simulink model "Hybrid_P2_Parallel"  (R2017b)
settings: Solver=FixedStepAuto  StartTime=0.0  StopTime=length(Speed)  FixedStep=0.01  MaxStep=0.01  RelTol=1e-3  EnableMultiTasking=on
PostLoadFcn:
  | , if any(exist('dsrtsu_mdlpostloadfcn', 'file') == [2, 3, 6]), try dsrtsu_mdlpostloadfcn('Execute', bdroot); catch fprintf('Error in PostLoadFcn (dsrtsu_mdlpostloadfcn) for model "%s":\n %s\n', bdroot, lasterr); end, end,
undefined symbols (not defined in the file): APP1_OOR, APP2_OOR, APP_Mismatch, Brk_Flt, cal, clt, Clutch, Clutch2, ClutchEngag, eng, Engine, EngOverTemp, ENGTRQ_MSMCH_Degraded_CP, ENGTRQ_MSMCH_ErrCritical_CP, ENGTRQ_MSMCH_LimpHome_CP, EngTrqMismatch, ess, ESSOverTemp, gb, KeyPos_Flt, LossCAN, MCUOverTemp, mot, MotDirMismatch, MotOverTemp, MotTrqMismatch, mph2kph, PRNDL_Flt, RegenFault, time, tloop
libraries: simulink x100, EC2_libraries x7, powerlib_meascontrol x2, lib_Actuators x1, CalculationGallon x1, lib_Chassis x1, autolibcoupling x1, autolibsharedcoupling x1, lib_DCDC x1, lib_Differential x1, lib_EMachine_2017a x1, lib_HVESS x1
(part 2 of 7)

== system Hybrid_P2_Parallel/Controller/HSC/Driver_Requests/APP_BPP to DrvIntndAxlTrq2 ==
  note: Note:Driver requested Axle Torque Calculation
  note: $Author: fy6949 $
      | $Rev: 577 $
      | $Date: 2017-1-19 08:53:15 -0500  $
  Sensors : Inport
  Diag : Inport  Port=2
  Controls : Inport  Port=3
  Bus Selector : BusSelector  OutputSignals=from_Analog.Driver_APP1,from_CAN.fromVEH_CAN.from_BCM.BrkPdlPos,from_CAN.fromEBCAN.from_ECM.VehSpdAvgDrvn,from_CAN.fromVEH_CAN.from_TCM.TrnGrRat,from_CAN.fromHV_CAN.from_MCU.INV_VCU_01.INV_Speed
  Bus Selector1 : BusSelector  OutputSignals=CompSig.RawSig.Driver_SigDiag.Drv_APP_Agree
  Bus Selector2 : BusSelector  OutputSignals=mode
  Post Driver Intnded Axle Torque : Subsystem
  Terminator : Terminator
  Terminator1 : Terminator
  IntndAxlTrq : Outport
  wires:
  Sensors/1 -> Bus Selector/1
  Controls/1 -> Bus Selector2/1
  Post Driver Intnded Axle Torque/1(IntndAxlTrq) -> IntndAxlTrq/1
  Bus Selector/2 -> Post Driver Intnded Axle Torque/2(BPP)  "<BrkPdlPos>"
  Bus Selector/3 -> Post Driver Intnded Axle Torque/3(VehicleSpeed)  "<VehSpdAvgDrvn>"
  Bus Selector/5 -> Post Driver Intnded Axle Torque/6(Motor_Speed)  "<INV_Speed>"
  Bus Selector/4 -> Post Driver Intnded Axle Torque/4(TransGearRatio)  "<TrnGrRat>"
  Bus Selector/1 -> Post Driver Intnded Axle Torque/1(APP)  "<Driver_APP1>"
  Post Driver Intnded Axle Torque/2(BrkIntndAxlTrq) -> Terminator/1
  Diag/1 -> Bus Selector1/1
  Bus Selector1/1 -> Terminator1/1  "<Drv_APP_Agree>"
  Bus Selector2/1 -> Post Driver Intnded Axle Torque/5(Mode)  "<mode>"

== system Hybrid_P2_Parallel/Controller/HSC/Powertrain Manager/Clutch Manager ==
  Sensors : Inport
  Control : Inport  Port=2
  Bus Creator : BusCreator  Inputs=2
  Bus Selector : BusSelector  OutputSignals=ClutchDisEngage
  Bus Selector1 : BusSelector  OutputSignals=from_CAN.fromEBCAN.from_CCU.CY01_posCurr,from_CAN.fromEBCAN.from_CCU.CY01_stMode,from_CAN.fromEBCAN.from_CCU.CY01_Counter,from_CAN.fromEBCAN.from_CCU.CY01_pCurr,from_CAN.fromHV_CAN.from_MCU.INV_VCU_01.INV_Speed,from_CAN.fromEBCAN.from_ECM.EngSpd,from_Analog.Driver_APP1,from_CAN.fromVEH_CAN.from_BCM.SysPwrMd,from_CAN.fromVEH_CAN.from_BCM.BrkPdlPos,from_CAN.fromVEH_CAN.from_TCM.TransEstGear
  Chart : Stateflow chart  Commented=on  TreatAsAtomicUnit=on
  Constant : Constant
  Constant1 : Constant  Value=2000
  Constant2 : Constant  Value=0
  Data Type Conversion : DataTypeConversion
  Switch : Switch  Criteria=u2 > Threshold
  Terminator{,1..9} (10 alike) : Terminator
  Out1 : Outport
  wires:
  Constant/1 -> Bus Creator/1  "MY15_CCU_stModeReq"
  Bus Creator/1 -> Out1/1
  Data Type Conversion/1 -> Bus Creator/2  "MY15_CCU_posDes"
  Control/1 -> Bus Selector/1
  Bus Selector/1 -> Switch/2  "<ClutchDisEngage>"
  Sensors/1 -> Bus Selector1/1
  Bus Selector1/1 -> Terminator/1  "<CY01_posCurr>"
  Bus Selector1/2 -> Terminator1/1  "<CY01_stMode>"
  Bus Selector1/3 -> Terminator2/1  "<CY01_Counter>"
  Bus Selector1/4 -> Terminator3/1  "<CY01_pCurr>"
  Bus Selector1/5 -> Terminator4/1  "<INV_Speed>"
  Bus Selector1/6 -> Terminator5/1  "<EngSpd>"
  Bus Selector1/7 -> Terminator6/1  "<Driver_APP1>"
  Bus Selector1/8 -> Terminator7/1  "<SysPwrMd>"
  Bus Selector1/9 -> Terminator8/1  "<BrkPdlPos>"
  Bus Selector1/10 -> Terminator9/1  "<TransEstGear>"
  Switch/1 -> Data Type Conversion/1
  Constant1/1 -> Switch/1
  Constant2/1 -> Switch/3

== system Hybrid_P2_Parallel/Controller/HSC/Powertrain Manager/HV Manager ==
  Sensors : Inport
  Controls : Inport  Port=2
  Axiomatic_Output_Manager : Subsystem
  BMS_Manager : Subsystem
  Bus Creator1 : BusCreator  Inputs=4
  DCDC Manager : Subsystem
  Invrter Manager : Subsystem
  OBC_Manager : Subsystem
  BMS_CAN : Outport
  HV_BUS_Status : Outport  Port=2
  OBC_CAN : Outport  Port=3
  OBC_Digital : Outport  Port=4
  BMS_Digital : Outport  Port=5
  Axiomatic_CAN : Outport  Port=6
  tag scope: MCU_CAN=global
  wires:
  Bus Creator1/1 -> [MCU_CAN]
  Invrter Manager/2(MCU_CAN) -> Bus Creator1/2  "MCU_CAN"
  Invrter Manager/1(MCU_Status) -> [MCU_Status], Bus Creator1/1  "MCU_Status"
  Sensors/1 -> BMS_Manager/1(Sensors), Invrter Manager/2(Sensors), DCDC Manager/1(BMSInput), Axiomatic_Output_Manager/1(Sensors), OBC_Manager/2(Sensors)
  [HV_BUS_Status] -> Invrter Manager/1(HV_Bus_Status)  "HV_BUS_Status"
  [HV_BUS_Status] -> Axiomatic_Output_Manager/2(HV_Bus_Status)
  BMS_Manager/2(HV_BUS_Status) -> [HV_BUS_Status], HV_BUS_Status/1  "HV_BUS_Status"
  [HV_BUS_Status] -> OBC_Manager/1(HV_Status)
  OBC_Manager/1(OBC CAN) -> OBC_CAN/1
  OBC_Manager/2(OBC_Digital) -> OBC_Digital/1
  Controls/1 -> BMS_Manager/2(Controls), Invrter Manager/3(Control), DCDC Manager/2(In1), DCDC Manager/3(In2)
  BMS_Manager/1(BMS CAN) -> BMS_CAN/1
  BMS_Manager/3(BMS Digital) -> BMS_Digital/1
  Axiomatic_Output_Manager/1(Axiomatic_CAN) -> Axiomatic_CAN/1
  Invrter Manager/3(MCU_Relay) -> Bus Creator1/3
  DCDC Manager/1(Out1) -> Bus Creator1/4
  [MCU_Status] -> BMS_Manager/3(In1)

== system Hybrid_P2_Parallel/Controller/HSC/Powertrain Manager/Output Conversion ==
  In1 : Inport
  In2 : Inport  Port=2
  In3 : Inport  Port=3
  In6 : Inport  Port=4
  In4 : Inport  Port=5
  In5 : Inport  Port=6
  In8 : Inport  Port=7
  In9 : Inport  Port=8
  In10 : Inport  Port=9
  In11 : Inport  Port=10
  Bus Creator : BusCreator  Inputs=14
  Bus Creator1 : BusCreator  Inputs=10
  Bus Selector2 : BusSelector  OutputSignals=powerMode,EnablePrplsn,ClutchDisEngage,EngAppReq,EngOnReq,MtrTrqCmd,EnableInverter,EngTrqCmd,HV_req,SysPwrMd_0_3,TransShftLvrPos,VehSpdAvgDrvn_kph,AccPos_Perc,SportsModeEnable
  Data Type Conversion{,2..3,5..13} (12 alike) : DataTypeConversion
  Memory : Memory
  Out1 : Outport
  wires:
  In10/1 -> Bus Creator1/9
  In9/1 -> Bus Creator1/8
  In8/1 -> Bus Creator1/7
  Memory/1 -> Data Type Conversion/1
  Data Type Conversion13/1 -> Bus Creator/13  "AccPos_Perc"
  Bus Selector2/13 -> Data Type Conversion13/1  "<AccPos_Perc>"
  Data Type Conversion12/1 -> Bus Creator/12  "VehSpdAvgDrvn_kph"
  Bus Selector2/12 -> Data Type Conversion12/1  "<VehSpdAvgDrvn_kph>"
  Data Type Conversion11/1 -> Bus Creator/11  "ShftLvrPos"
  Bus Selector2/11 -> Data Type Conversion11/1  "<TransShftLvrPos>"
  In5/1 -> Bus Creator1/6
  Bus Creator/1 -> Bus Creator1/5  "Controls"
  In3/1 -> Bus Creator1/3
  In2/1 -> Bus Creator1/2
  In1/1 -> Bus Creator1/1
  Bus Creator1/1 -> Out1/1
  Data Type Conversion5/1 -> Bus Creator/5  "EngOnReq"
  Data Type Conversion/1 -> Bus Creator/1  "powerMode"
  Data Type Conversion10/1 -> Bus Creator/10  "SysPwrMd"
  Data Type Conversion9/1 -> Bus Creator/9  "HV_req"
  Data Type Conversion8/1 -> Bus Creator/8  "EngTrqCmd"
  Data Type Conversion7/1 -> Bus Creator/7  "Inverter_Enable"
  Data Type Conversion6/1 -> Bus Creator/6  "Torque_Command"
  Bus Selector2/4 -> Bus Creator/4  "<EngAppReq>"
  Data Type Conversion3/1 -> Bus Creator/3  "ClutchDisEngage"
  Data Type Conversion2/1 -> Bus Creator/2  "EnablePrplsn"
  Bus Selector2/10 -> Data Type Conversion10/1  "<SysPwrMd_0_3>"
  Bus Selector2/9 -> Data Type Conversion9/1  "<HV_req>"
  Bus Selector2/8 -> Data Type Conversion8/1  "<EngTrqCmd>"
  Bus Selector2/7 -> Data Type Conversion7/1  "<EnableInverter>"
  Bus Selector2/6 -> Data Type Conversion6/1  "<MtrTrqCmd>"
  Bus Selector2/5 -> Data Type Conversion5/1  "<EngOnReq>"
  Bus Selector2/3 -> Data Type Conversion3/1  "<ClutchDisEngage>"
  Bus Selector2/2 -> Data Type Conversion2/1  "<EnablePrplsn>"
  Bus Selector2/1 -> Memory/1  "<powerMode>"
  In4/1 -> Bus Selector2/1
  In11/1 -> Bus Creator1/10
  Bus Selector2/14 -> Bus Creator/14  "<SportsModeEnable>"
  In6/1 -> Bus Creator1/4

== system Hybrid_P2_Parallel/Controller/HSC/Powertrain Manager/Thermal Manager ==
  In2 : Inport
  Bus Creator : BusCreator  Inputs=3
  Bus Creator1 : BusCreator  Inputs=4
  Bus Creator2 : BusCreator  Inputs=4
  Bus Creator3 : BusCreator  Inputs=3
  Bus Creator4 : BusCreator  Inputs=1
  Bus Selector : BusSelector  OutputSignals=from_CAN.fromEBCAN.from_ECM.EngCltTmp,from_CAN.fromHV_CAN.from_BMSHybrid.BMS_Temperatur,from_CAN.fromHV_CAN.from_MCU.INV_VCU_04.INV_InverterTemperature,from_CAN.fromHV_CAN.from_MCU.INV_VCU_04.INV_ElectricMachineTemperature,from_CAN.fromEBCAN.from_ECM.EngRunAtv,from_CAN.fromHV_CAN.from_BMSHybrid.BMS_HYB_02.BMS_IstModus,from_CAN.fromVEH_CAN.from_BCM.SysPwrMd,from_CAN.fromEBCAN.from_ECM.VehSpdAvgDrvn
  Bus Selector3 : BusSelector  OutputSignals=from_CAN.fromHV_CAN.from_BMSHybrid.BMS_HYB_02.BMS_Fehler_Pilot
  Compare To Constant1 : simulink/Logic and Bit Operations/Compare To Constant  relop=>  const=0  OutDataTypeStr=boolean
  Cooling Fan Manger : Subsystem
  Data Type Conversion : DataTypeConversion  OutDataTypeStr=double
  ESS Pump Manger : Subsystem
  MotInv Pump Manger : Subsystem
  Out1 : Outport
  wires:
  Bus Selector/8 -> Bus Creator/3  "<VehSpdAvgDrvn>"
  Bus Selector/7 -> Bus Creator3/3  "<SysPwrMd>"
  Bus Selector/6 -> Bus Creator3/2  "<BMS_IstModus>"
  Bus Selector/5 -> Bus Creator3/1  "<EngRunAtv>"
  Bus Selector/4 -> Bus Creator2/4  "<INV_ElectricMachineTemperature>"
  Bus Selector/3 -> Bus Creator2/3  "<INV_InverterTemperature>"
  Bus Selector/2 -> Bus Creator2/2  "<BMS_Temperatur>"
  Bus Selector/1 -> Bus Creator2/1  "<EngCltTmp>"
  Bus Creator1/1 -> Out1/1  "Thermal_Control"
  Cooling Fan Manger/1(Fan_control) -> Bus Creator1/1  "Fan_Control"
  Bus Creator/1 -> Cooling Fan Manger/1(Temp), ESS Pump Manger/1(ESS_temp), MotInv Pump Manger/1(MotInv_temp)
  ESS Pump Manger/1(ESS_Thermal_Control) -> Bus Creator1/2  "ESS_Pump_Control"
  MotInv Pump Manger/1(MotInvpump_control) -> Bus Creator1/3  "MotMCU_Pump_Control"
  Bus Creator2/1 -> Bus Creator/1  "Temp_Signals"
  Bus Creator3/1 -> Bus Creator/2  "Component_State"
  In2/1 -> Bus Selector3/1, Bus Selector/1
  Bus Selector3/1 -> Compare To Constant1/1  "<BMS_Fehler_Pilot>"
  Bus Creator4/1 -> Bus Creator1/4  "Pump_Commands"
  Data Type Conversion/1 -> Bus Creator4/1  "FuelPump_Disable"
  Compare To Constant1/1 -> Data Type Conversion/1

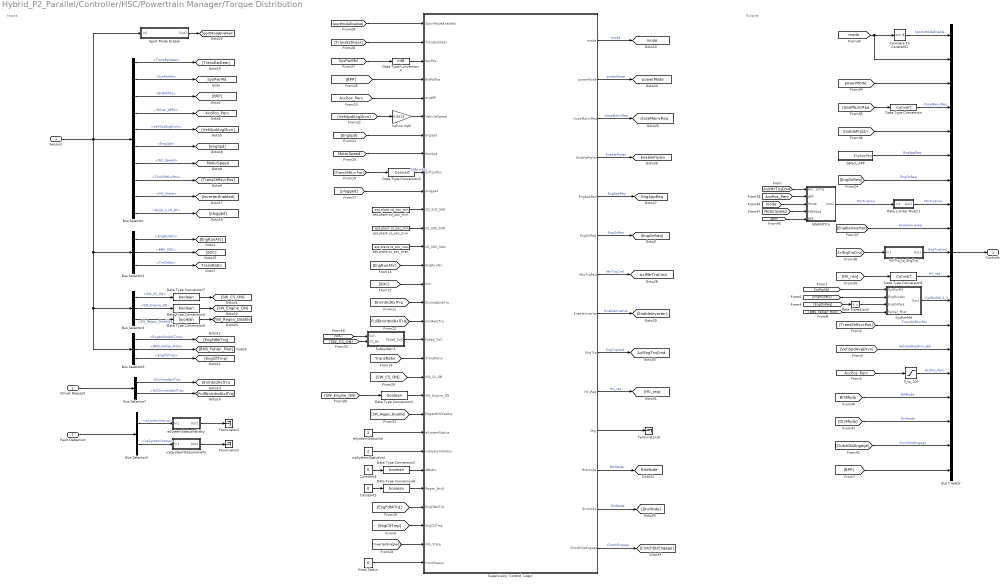
== system Hybrid_P2_Parallel/Controller/HSC/Powertrain Manager/Torque Distribution ==
  note: Inputs
  note: Outputs
  Sensors : Inport
  Driver Request : Inport  Port=2
  Fault Detection : Inport  Port=3
  0_to_100 : Saturate  UpperLimit=100  LowerLimit=0
  AxlTrq_to_EngTrq : Subsystem
  Bus Creator : BusCreator  Inputs=19
  Bus Selector : BusSelector  OutputSignals=from_CAN.fromVEH_CAN.from_TCM.TransEstGear,from_CAN.fromVEH_CAN.from_BCM.SysPwrMd,from_CAN.fromVEH_CAN.from_BCM.BrkPdlPos,from_Analog.Driver_APP1,from_CAN.fromEBCAN.from_ECM.VehSpdAvgDrvn,from_CAN.fromEBCAN.from_ECM.EngSpd,from_CAN.fromHV_CAN.from_MCU.INV_VCU_01.INV_Speed,from_CAN.fromVEH_CAN.from_TCM.TrnsShftLvrPos,from_CAN.fromHV_CAN.from_MCU.INV_VCU_01.INV_State,from_CAN.fromHV_CAN.from_OBC.NLG5_ST.NLG5_S_CP_DT
  Bus Selector1 : BusSelector  OutputSignals=from_CAN.fromEBCAN.from_ECM.EngRunAtv,from_CAN.fromHV_CAN.from_BMSHybrid.BMS_SOC,from_CAN.fromVEH_CAN.from_TCM.TrnGrRat
  Bus Selector2 : BusSelector  OutputSignals=eSystemDiagOut.eSystemStatus,iceSystemDiagOut.iceSystemStatus
  Bus Selector4 : BusSelector  OutputSignals=from_Digital.SW_CS_ON,from_Digital.SW_Engine_ON,from_Digital.SW_Regen_Disable
  Bus Selector6 : BusSelector  OutputSignals=from_CAN.fromEBCAN.from_ECM.EngActStdyStTorq,from_CAN.fromHV_CAN.from_BMSHybrid.BMS_HYB_02.BMS_Fehler_Pilot,from_CAN.fromEBCAN.from_ECM.EngCltTmp
  Bus Selector7 : BusSelector  OutputSignals=DrvIntndAxlTrq,FullDrvIntndAxlTrq
  Compare To Constant1 : simulink/Logic and Bit Operations/Compare To Constant  relop===  const=4  OutDataTypeStr=boolean
  Constant2 : Constant  Value=0
  Constant3 : Constant  Value=0
  Data Type Conversion : DataTypeConversion
  Data Type Conversion{1..2,5..8} (6 alike) : DataTypeConversion  OutDataTypeStr=boolean
  Data Type Conversion3 : DataTypeConversion
  Data Type Conversion4 : DataTypeConversion  OutDataTypeStr=int8
  Data Type Conversion9 : DataTypeConversion
  Hood Status : Constant  Value=0
  IdleMotTrq : Subsystem
  Rate Limiter Motor1 : Subsystem
  Rate Transition3 : RateTransition
  Select_APP : Subsystem
  Sport Mode Enable : Subsystem
  Subsystem1 : Subsystem
  Supervisory  Control  Logic : Stateflow chart  TreatAsAtomicUnit=on
  SysPwrMd : Subsystem
  Terminator1 : Terminator
  Terminator10 : Terminator
  Terminator2 : Terminator
  eSystemStatusVal : Constant  Value=2
  eSystemStatusValidity : Subsystem
  ess.plant.cd_soc_min : Constant  Value=ess.plant.cd_soc_min
  ess.plant.cs_soc_max : Constant  Value=ess.plant.cs_soc_max
  ess.plant.cs_soc_min : Constant  Value=ess.plant.cs_soc_min
  iceSystemStatusVal : Constant  Value=2
  iceSystemStatusValidity : Subsystem
  kph to mph : Gain  Gain=0.6213
  Controls : Outport
  tag scope: AccPos_Perc=global, AxlEngTrqCmd=global, AxlMtrTrqCmd=global, BrkMode=global, DrvIntndAxlTrq=global, EnablePrplsn=global, EngAppReq=global, MotorSpeed=global, SportModeEnabled=global, SysPwrMd=global, TransRatio=global, closeMaincReq=global, mode=global, powerMode=global
  wires:
  [AxlMtrTrqCmd] -> IdleMotTrq/1(AxlMotTrq)
  [MotorSpeed] -> IdleMotTrq/4(FdbkSpd)
  Hood Status/1 -> Supervisory  Control  Logic/30(HoodStatus)
  [plugged] -> Supervisory  Control  Logic/10(plugged)
  AxlTrq_to_EngTrq/1(Out1) -> Bus Creator/10  "EngTrqCmd"
  [closeMaincReq] -> Data Type Conversion/1
  Compare To Constant1/1 -> Bus Creator/1  "SportsModeEnable"
  [EngRunAtv] -> SysPwrMd/2(EngRunAtv)
  [ClutchDisEngage] -> Bus Creator/18  "ClutchDisEngage"
  [BPP] -> Bus Creator/19
  [AxlEngTrqCmd] -> AxlTrq_to_EngTrq/1(In1)
  [mode] -> Compare To Constant1/1, Bus Creator/2
  [TransShftLvrPos] -> Bus Creator/13  "TransShftLvrPos"
  [DrvMode] -> Bus Creator/17  "DrvMode"
  [SysPwrMd] -> SysPwrMd/1(SysPwrMd)
  SysPwrMd/1(Out1) -> Bus Creator/12  "SysPwrMd_0_3"
  [VehSpdAvgDrvn] -> Bus Creator/14  "VehSpdAvgDrvn_kph"
  Data Type Conversion9/1 -> Bus Creator/11  "HV_req"
  [BMS_Fehler_Pilot] -> SysPwrMd/4(Fehler_Pilot)
  [EnablePrplsn] -> Bus Creator/5
  [AccPos_Perc] -> 0_to_100/1
  [EnableInverter] -> Bus Creator/9  "EnableInverter"
  [EngOnReq] -> Bus Creator/7  "EngOnReq"
  [HV_req] -> Data Type Conversion9/1
  Select_APP/1(EngAppReq) -> Bus Creator/6  "EngAppReq"
  [BrkMode] -> Bus Creator/16  "BrkMode"
  0_to_100/1 -> Bus Creator/15  "AccPos_Perc"
  [powerMode] -> Bus Creator/3
  Data Type Conversion/1 -> Bus Creator/4  "closeMaincReq"
  [EngOnReq] -> Rate Transition3/1
  Rate Transition3/1 -> SysPwrMd/3(EngOnReq)
  Bus Creator/1 -> Controls/1
  Sensors/1 -> Bus Selector/1, Bus Selector1/1, Bus Selector4/1, Bus Selector6/1, Sport Mode Enable/1(In1)
  Bus Selector/1 -> [TransEstGear]  "<TransEstGear>"
  Bus Selector/2 -> [SysPwrMd]  "<SysPwrMd>"
  Bus Selector/3 -> [BPP]  "<BrkPdlPos>"
  Bus Selector/4 -> [AccPos_Perc]  "<Driver_APP1>"
  Bus Selector/5 -> [VehSpdAvgDrvn]  "<VehSpdAvgDrvn>"
  Bus Selector/6 -> [EngSpd]  "<EngSpd>"
  Bus Selector/7 -> [MotorSpeed]  "<INV_Speed>"
  Bus Selector/9 -> [InverterEnabled]  "<INV_State>"
  Bus Selector1/1 -> [EngRunAtv]  "<EngRunAtv>"
  Bus Selector/8 -> [TransShftLvrPos]  "<TrnsShftLvrPos>"
  Bus Selector1/3 -> [TransRatio]  "<TrnGrRat>"
  Fault Detection/1 -> Bus Selector2/1
  Bus Selector2/1 -> eSystemStatusValidity/1(In1)  "<eSystemStatus>"
  Bus Selector2/2 -> iceSystemStatusValidity/1(In1)  "<iceSystemStatus>"
  Bus Selector4/3 -> Data Type Conversion6/1  "<SW_Regen_Disable>"
  Bus Selector4/1 -> Data Type Conversion7/1  "<SW_CS_ON>"
  Bus Selector4/2 -> Data Type Conversion5/1  "<SW_Engine_ON>"
  eSystemStatusValidity/1(Out1) -> Terminator1/1
  iceSystemStatusValidity/1(Out1) -> Terminator2/1
  Bus Selector/10 -> [plugged]  "<NLG5_S_CP_DT>"
  Data Type Conversion5/1 -> [SW_Engine_ON]
  Data Type Conversion6/1 -> [SW_Regen_Disable]
  Bus Selector6/1 -> [EngFdbkTrq]  "<EngActStdyStTorq>"
  Bus Selector6/2 -> [BMS_Fehler_Pilot]  "<BMS_Fehler_Pilot>"
  Bus Selector6/3 -> [EngCltTmp]  "<EngCltTmp>"
  Bus Selector7/2 -> [FullDrvIntndAxlTrq]  "<FullDrvIntndAxlTrq>"
  Sport Mode Enable/1(Out1) -> [SportModeEnabled]
  Bus Selector1/2 -> [SOC]  "<BMS_SOC>"
  Data Type Conversion7/1 -> [SW_CS_ON]
  Driver Request/1 -> Bus Selector7/1
  Bus Selector7/1 -> [DrvIntndAxlTrq]  "<DrvIntndAxlTrq>"
  Supervisory  Control  Logic/14(ClutchDisEngage) -> [ClutchDisEngage]  "ClutchEngage"
  Supervisory  Control  Logic/13(Drvmode) -> [DrvMode]  "DrvMode"
  Supervisory  Control  Logic/10(HV_Req) -> [HV_req]  "HV_req"
  Supervisory  Control  Logic/9(EngTrq) -> [AxlEngTrqCmd]  "EngTrqCmd"
  Supervisory  Control  Logic/7(MotTrqReq) -> [AxlMtrTrqCmd]  "MtrTrqCmd"
  Supervisory  Control  Logic/6(EngOnReq) -> [EngOnReq]  "EngOnReq"
  [SW_CS_ON] -> Subsystem1/2(CS_On)
  [SW_Regen_Disable] -> Supervisory  Control  Logic/22(RegenBrkDisable)
  [SW_CS_ON] -> Supervisory  Control  Logic/20(SW_CS_ON)
  [SportModeEnabled] -> Supervisory  Control  Logic/1(SportModeEnabled)
  Data Type Conversion4/1 -> Supervisory  Control  Logic/3(KeyPos)
  [SysPwrMd] -> Data Type Conversion4/1
  [TransEstGear] -> Supervisory  Control  Logic/2(TransEstGear)
  [BPP] -> Supervisory  Control  Logic/4(BrkPdlPos)
  [AccPos_Perc] -> Supervisory  Control  Logic/5(drvAPP)
  [VehSpdAvgDrvn] -> kph to mph/1
  [EngSpd] -> Supervisory  Control  Logic/7(EngSpd)
  [TransShftLvrPos] -> Data Type Conversion3/1
  [SOC] -> Subsystem1/1(SoC)
  [SOC] -> Supervisory  Control  Logic/15(SoC)
  [TransRatio] -> Supervisory  Control  Logic/19(TransRatio)
  [EngRunAtv] -> Supervisory  Control  Logic/14(EngRunAtv)
  [EngFdbkTrq] -> Supervisory  Control  Logic/27(EngFdbkTrq)
  [EngCltTmp] -> Supervisory  Control  Logic/28(EngCtlTmp)
  Supervisory  Control  Logic/5(EngAppReq) -> [EngAppReq]  "EngAppReq"
  eSystemStatusVal/1 -> Supervisory  Control  Logic/23(eSystemStatus)
  iceSystemStatusVal/1 -> Supervisory  Control  Logic/24(iceSystemStatus)
  Data Type Conversion8/1 -> Supervisory  Control  Logic/26(Regen_fault)
  Supervisory  Control  Logic/12(Brkmode) -> [BrkMode]  "BrkMode"
  Subsystem1/1(Faked_SoC) -> Supervisory  Control  Logic/18(Faked_SoC)
  Data Type Conversion1/1 -> Supervisory  Control  Logic/25(ABSAtv)
  Constant3/1 -> Data Type Conversion1/1
  [FullDrvIntndAxlTrq] -> Supervisory  Control  Logic/17(IntdAxleTrq)
  [DrvIntndAxlTrq] -> Supervisory  Control  Logic/16(DrvIntdAxleTrq)
  Supervisory  Control  Logic/11(Chg) -> Terminator10/1
  Constant2/1 -> Data Type Conversion8/1
  kph to mph/1 -> Supervisory  Control  Logic/6(VehicleSpeed)
  Data Type Conversion3/1 -> Supervisory  Control  Logic/9(ShftLvrPos)  "ShftLvrPos"
  Supervisory  Control  Logic/1(mode) -> [mode]  "mode"
  Supervisory  Control  Logic/2(powerMode) -> [powerMode]  "powerMode"
  Supervisory  Control  Logic/3(closeMaincReq) -> [closeMaincReq]  "closeMaincReq"
  Supervisory  Control  Logic/4(EnablePrplsn) -> [EnablePrplsn]  "EnablePrplsn"
  Supervisory  Control  Logic/8(EnableInverter) -> [EnableInverter]  "EnableInverter"
  ess.plant.cs_soc_max/1 -> Supervisory  Control  Logic/13(CS_SOC_MAX)
  ess.plant.cs_soc_min/1 -> Supervisory  Control  Logic/12(CS_SOC_MIN)
  ess.plant.cd_soc_min/1 -> Supervisory  Control  Logic/11(CD_SOC_MIN)
  [SW_Engine_ON] -> Data Type Conversion2/1
  Data Type Conversion2/1 -> Supervisory  Control  Logic/21(SW_Engine_ON)
  [InverterEnabled] -> Supervisory  Control  Logic/29(INV_State)
  IdleMotTrq/1(Out1) -> Rate Limiter Motor1/1(In1)  "MtrTrqCmd"
  Rate Limiter Motor1/1(Out1) -> Bus Creator/8  "MtrTrqCmd"
  [AccPos_Perc] -> IdleMotTrq/2(APP)
  [mode] -> IdleMotTrq/3(Mode)
  [BPP] -> IdleMotTrq/5(BPP)
  [MotorSpeed] -> Supervisory  Control  Logic/8(MotSpd)

== system Hybrid_P2_Parallel/Controller/HSC/Camaro Fault Detection/Component Diagnostic/Driver Input Diagnostic ==
  note: APP1
      | APP2
      | BPP
      | Driver Component Status
      |
      | 1
      | 1
      | 1
      | 1
      |
      | 0
      | 1
      | 1
      | 1
      |
      | 1
      | 0
      | 1
      | 1
      |
      | 0
      | 0
      | 1
      | 0
      |
      | 1
      | 1
      | 0
      | 0
      |
      | 0
      | 0
      | 0
      | 0
  note: Driver_CompStatus
      | 1 = Component Online
      | 0 = Component Offline
  In1 : Inport
  Bus Selector : BusSelector  OutputSignals=Driver_SigDiag.Drv_APP1_[%]_SigValid,Driver_SigDiag.Drv_APP2_[%]_SigValid,Driver_SigDiag.Drv_APP_Agree,Driver_SigDiag.Drv_BPP_[%]_SigValid,Driver_SigDiag.Drv_KeyPos_[0 3]_SigValid,Driver_SigDiag.Drv_PRNDL_SigValid,Driver_SigDiag.Brake_Failed
  Driver_Input_Diag : Stateflow chart  TreatAsAtomicUnit=on
  Logical Operator : Logic  Inputs=3  AllPortsSameDT=off  OutDataTypeStr=boolean
  Out1 : Outport
  wires:
  Bus Selector/7 -> Driver_Input_Diag/5(BrakeFail)  "<Brake_Failed>"
  Bus Selector/6 -> Driver_Input_Diag/4(PRNDL)  "<Drv_PRNDL_SigValid>"
  Bus Selector/5 -> Driver_Input_Diag/3(KeyPos)  "<Drv_KeyPos_[0 3]_SigValid>"
  Bus Selector/3 -> Logical Operator/3  "<Drv_APP_Agree>"
  Logical Operator/1 -> Driver_Input_Diag/1(APP_Valid)  "APP_Valid"
  Driver_Input_Diag/1(Driver_Input_Status) -> Out1/1  "Driver_Input_Status"
  Bus Selector/4 -> Driver_Input_Diag/2(Drv_BPP_SigValid)  "<Drv_BPP_[%]_SigValid>"
  Bus Selector/2 -> Logical Operator/2  "<Drv_APP2_[%]_SigValid>"
  Bus Selector/1 -> Logical Operator/1  "<Drv_APP1_[%]_SigValid>"
  In1/1 -> Bus Selector/1

== system Hybrid_P2_Parallel/Controller/HSC/Camaro Fault Detection/Component Diagnostic/ESS Component Diagnostic ==
  note: (Need modify)
  In1 : Inport
  BMS_CompDiag1 : Stateflow chart  TreatAsAtomicUnit=on
  Bus Selector : BusSelector  OutputSignals=ESS_SigDiag.BMS_RollingAliveActive_SigValid,ESS_SigDiag.BMS_contactorsFailed_Detected,ESS_SigDiag.BMS_essTemp_[degC]_SigValid,ESS_SigDiag.essTempRange[0_4],ESS_SigDiag.BMS_essSOC_0_1_SigValid,ESS_SigDiag.essTempRange[0_4],ESS_SigDiag.essCur_A_SigValid,ESS_SigDiag.BMSgdf_SigValid,Driver_SigDiag.Drv_KeyPos_[0 3]_SigValid
  Compare To Zero : simulink/Logic and Bit Operations/Compare To Zero  relop===  OutDataTypeStr=boolean
  Data Type Conversion : DataTypeConversion
  HVessFltReset : Constant
  Logical Operator : Logic  Operator=OR  AllPortsSameDT=off  OutDataTypeStr=boolean
  Logical Operator1 : Logic  AllPortsSameDT=off  OutDataTypeStr=boolean
  Terminator : Terminator
  Terminator1 : Terminator
  Out1 : Outport
  wires:
  [contactorsFailed_Detected] -> Logical Operator1/1
  Logical Operator1/1 -> BMS_CompDiag1/6(ess_GroundFault)
  Bus Selector/8 -> Logical Operator1/2  "<BMSgdf_SigValid>"
  Logical Operator/1 -> BMS_CompDiag1/7(ClearFault)
  HVessFltReset/1 -> Logical Operator/2
  Compare To Zero/1 -> Logical Operator/1
  Bus Selector/9 -> Compare To Zero/1  "<Drv_KeyPos_[0 3]_SigValid>"
  Bus Selector/7 -> BMS_CompDiag1/5(essCur_A_SigValid)  "<essCur_A_SigValid>"
  Bus Selector/6 -> Terminator1/1  "<essTempRange[0_4]>"
  Bus Selector/5 -> BMS_CompDiag1/4(BMS_essSOC_0_1_SigValid)  "<BMS_essSOC_0_1_SigValid>"
  Data Type Conversion/1 -> BMS_CompDiag1/3(BMS_essTemp_SigValid)  "BMS_essTemp_SigValid"
  Bus Selector/3 -> Data Type Conversion/1  "<BMS_essTemp_[degC]_SigValid>"
  Bus Selector/4 -> Terminator/1  "<essTempRange[0_4]>"
  BMS_CompDiag1/1(BMS_Status) -> Out1/1  "BMS_Status"
  Bus Selector/2 -> BMS_CompDiag1/2(BMS_contactorsFailed_SigValid), [contactorsFailed_Detected]  "<BMS_contactorsFailed_Detected>"
  Bus Selector/1 -> BMS_CompDiag1/1(BMS_RollingAliveActive_SigValid)  "<BMS_RollingAliveActive_SigValid>"
  In1/1 -> Bus Selector/1

== system Hybrid_P2_Parallel/Controller/HSC/Camaro Fault Detection/Component Diagnostic/Engine Component Diagnostic ==
  note: Notes
  note: 0: component needs to be offline
      | 1: component needs torque plant to deliver creep torque
      | 2: component needs torque plant to limit maximum torque delivery
      | 3: component needs torque plant to operate normally
  note: add the temperature, mismatch torquesignal and have different status to the component
  note: Eng_tempRange
      | 1: normal
      | 2: high range
      | 3:above max
  note: ENGTRQ_MSMCH_Degraded_CP (40Nm): ENGTRQ_Degraded fault code.
      | ENGTRQ_MSMCH_LimpHome_CP (70Nm): ENGTRQ_LimpHome
      | ENGTRQ_MSMCH_ErrCritical_CP (100Nm): ENGTRQ_ErrCritical
  note: Eng_Torq_MsmchLevel
      | 1:Normal torque
      | 2: Limit max power
      | 3: Deliver creep torque
      | 4: offline
  In1 : Inport
  Bus Selector : BusSelector  OutputSignals=Engine_SigDiag.ECMRollingAliveActive,Engine_SigDiag.engTrqCmdRecvd_SigValid,Engine_SigDiag.ECMTrqCmd_Nm,Engine_SigDiag.EngActStdyStTorq_Nm,Engine_SigDiag.EngRunAtValid,Engine_SigDiag.Engine_Speed_rpm_SigValid,Engine_SigDiag.Eng_TempValid,Engine_SigDiag.Eng_TempRange[123],Driver_SigDiag.Drv_KeyPos_[0 3]_SigValid
  Bus Selector1 : BusSelector  OutputSignals=Eng_Torque_Mismch_Critical
  Compare To Zero : simulink/Logic and Bit Operations/Compare To Zero  relop===  OutDataTypeStr=boolean
  ECM_CompDiag : Stateflow chart  TreatAsAtomicUnit=on
  Eng_FltReset : Constant
  Eng_Torq_MsmchLevel : Stateflow chart  Commented=on  TreatAsAtomicUnit=on
  Logical Operator : Logic  Operator=OR  AllPortsSameDT=off  OutDataTypeStr=boolean
  Override  engTrqCmd : Subsystem
  Terminator1 : Terminator
  TorqMismatch Detection : Subsystem
  Out1 : Outport
  Out2 : Outport  Port=2
  wires:
  Override  engTrqCmd/1(Out1) -> ECM_CompDiag/2(engTrqCmdRecvd_SigValid)
  Bus Selector1/1 -> ECM_CompDiag/3(Eng_Torq_Msmch)  "<Eng_Torque_Mismch_Critical>"
  TorqMismatch Detection/1(Eng_Torque_Mismch) -> Out2/1, Bus Selector1/1  "EngTrqMismchType"
  Bus Selector/5 -> TorqMismatch Detection/3(In3)  "<EngRunAtValid>"
  Bus Selector/4 -> TorqMismatch Detection/2(In2)  "<EngActStdyStTorq_Nm>"
  Bus Selector/3 -> TorqMismatch Detection/1(In1)  "<ECMTrqCmd_Nm>"
  Bus Selector/8 -> ECM_CompDiag/5(Eng_TempRange_123)  "<Eng_TempRange[123]>"
  Bus Selector/7 -> Terminator1/1  "<Eng_TempValid>"
  Bus Selector/9 -> Compare To Zero/1  "<Drv_KeyPos_[0 3]_SigValid>"
  Logical Operator/1 -> ECM_CompDiag/6(ClearFault)
  Eng_FltReset/1 -> Logical Operator/2
  Compare To Zero/1 -> Logical Operator/1
  ECM_CompDiag/1(ECM_Status) -> Out1/1  "ECM_Status"
  Bus Selector/6 -> ECM_CompDiag/4(Engine_Speed_rpm_SigValid)  "<Engine_Speed_rpm_SigValid>"
  Bus Selector/2 -> Override  engTrqCmd/1(In1)  "<engTrqCmdRecvd_SigValid>"
  Bus Selector/1 -> ECM_CompDiag/1(ECM_RollingAliveActive)  "<ECMRollingAliveActive>"
  In1/1 -> Bus Selector/1

== system Hybrid_P2_Parallel/Controller/HSC/Camaro Fault Detection/Component Diagnostic/Override Driver Status ==
  note: Override Switch Subsystem
  note: This subsystem is used to override the model value of a signal to a constant value
  In1 : Inport
  Data Type Conversion3 : DataTypeConversion
  Override Value : Constant  OutDataTypeStr=double
  Override_Driver_Status : Constant  Value=0
  Switch : Switch  Criteria=u2 > Threshold
  Out1 : Outport
  wires:
  Data Type Conversion3/1 -> Switch/3
  Override Value/1 -> Switch/1
  Switch/1 -> Out1/1
  In1/1 -> Data Type Conversion3/1
  Override_Driver_Status/1 -> Switch/2

== system Hybrid_P2_Parallel/Controller/HSC/Camaro Fault Detection/Component Diagnostic/Override ESS Status ==
  note: Override Switch Subsystem
  note: This subsystem is used to override the model value of a signal to a constant value
  In1 : Inport
  Data Type Conversion3 : DataTypeConversion
  Override Value : Constant  Value=2  OutDataTypeStr=double
  Override_ESS_Status : Constant  Value=0
  Switch : Switch  Criteria=u2 > Threshold
  Terminator : Terminator
  Out1 : Outport
  wires:
  Data Type Conversion3/1 -> Switch/3
  Override Value/1 -> Switch/1, Out1/1
  Override_ESS_Status/1 -> Switch/2
  In1/1 -> Data Type Conversion3/1
  Switch/1 -> Terminator/1

== system Hybrid_P2_Parallel/Controller/HSC/Camaro Fault Detection/Component Diagnostic/Override Engine Status ==
  note: Override Switch Subsystem
  note: This subsystem is used to override the model value of a signal to a constant value
  In1 : Inport
  Data Type Conversion3 : DataTypeConversion
  Override Value1 : Constant  Value=2  OutDataTypeStr=double
  Override_Engine_Status : Constant  Value=0
  Switch : Switch  Criteria=u2 > Threshold
  Terminator : Terminator
  Out1 : Outport
  wires:
  Data Type Conversion3/1 -> Switch/3
  Override_Engine_Status/1 -> Switch/2
  Override Value1/1 -> Switch/1, Out1/1
  In1/1 -> Data Type Conversion3/1
  Switch/1 -> Terminator/1

== system Hybrid_P2_Parallel/Controller/HSC/Camaro Fault Detection/Component Diagnostic/Override TCM Status ==
  note: Override Switch Subsystem
  note: This subsystem is used to override the model value of a signal to a constant value
  In1 : Inport
  Data Type Conversion3 : DataTypeConversion
  Override Value1 : Constant  Value=2  OutDataTypeStr=double
  Override_TCM_Status : Constant  Value=0
  Switch : Switch  Criteria=u2 > Threshold
  Out1 : Outport
  wires:
  Data Type Conversion3/1 -> Switch/3
  Override Value1/1 -> Switch/1
  Override_TCM_Status/1 -> Switch/2
  Switch/1 -> Out1/1
  In1/1 -> Data Type Conversion3/1

== system Hybrid_P2_Parallel/Controller/HSC/Camaro Fault Detection/Component Diagnostic/Transmission Component Diagnostic ==
  In1 : Inport
  Bus Selector : BusSelector  OutputSignals=Transmission_SigDiag.TCMRollingAliveActive_SigValid,Transmission_SigDiag.LvrPosTrnsShft_SigValid,Transmission_SigDiag.TransEstGear_SigValid,Transmission_SigDiag.LockupCmd_SigValid,Transmission_SigDiag.VehDirFault
  TCM_CompDia : Stateflow chart  TreatAsAtomicUnit=on
  Out1 : Outport
  wires:
  Bus Selector/5 -> TCM_CompDia/5(VehDirFault)  "<VehDirFault>"
  TCM_CompDia/1(TCM_Status) -> Out1/1  "TCM_Status"
  Bus Selector/4 -> TCM_CompDia/4(LockupCmd_SigValid)  "<LockupCmd_SigValid>"
  Bus Selector/3 -> TCM_CompDia/3(TransEstGear_SigValid)  "<TransEstGear_SigValid>"
  Bus Selector/2 -> TCM_CompDia/2(LvrPosTrnsShft_SigValid)  "<LvrPosTrnsShft_SigValid>"
  Bus Selector/1 -> TCM_CompDia/1(TCMRollingAliveActive_SigValid)  "<TCMRollingAliveActive_SigValid>"
  In1/1 -> Bus Selector/1

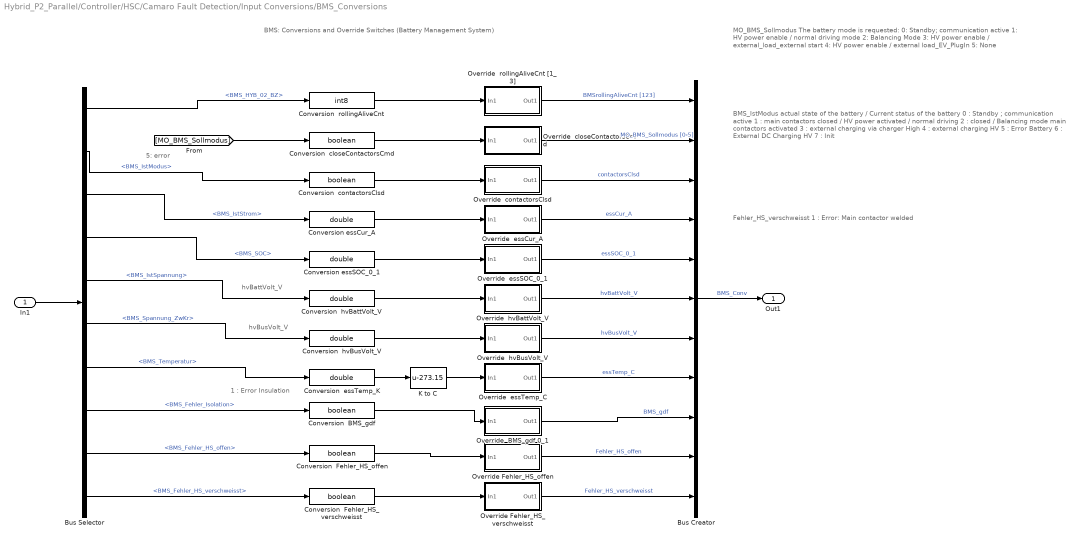
== system Hybrid_P2_Parallel/Controller/HSC/Camaro Fault Detection/Input Conversions/BMS_Conversions ==
  note: BMS: Conversions and Override Switches
      | (Battery Management System)
  note: hvBattVolt_V
  note: hvBusVolt_V
  note: 5: error
  note: 1 : Error Insulation
  note: MO_BMS_Sollmodus
      | The battery mode is requested:
      | 0: Standby; communication active
      | 1: HV power enable / normal driving mode
      | 2: Balancing Mode
      | 3: HV power enable / external_load_external start
      | 4: HV power enable / external load_EV_PlugIn
      | 5: None
  note: BMS_IstModus
      | actual state of the battery / Current status of the battery
      | 0 : Standby ; communication active
      | 1 : main contactors closed / HV power activated / normal driving
      | 2 : closed / Balancing mode main contactors activated
      | 3 : external charging via charger High
      | 4 : external charging HV
      | 5 : Error Battery
      | 6 : External DC Charging HV
      | 7 : Init
  note: Fehler_HS_verschweisst
      | 1 : Error: Main contactor welded
  In1 : Inport
  Bus Creator : BusCreator  Inputs=11
  Bus Selector : BusSelector  OutputSignals=from_CAN.fromHV_CAN.from_BMSHybrid.BMS_HYB_02.BMS_HYB_02_BZ,from_CAN.fromHV_CAN.from_BMSHybrid.BMS_HYB_02.BMS_IstModus,from_CAN.fromHV_CAN.from_BMSHybrid.BMS_HYB_02.BMS_IstStrom,from_CAN.fromHV_CAN.from_BMSHybrid.BMS_SOC,from_CAN.fromHV_CAN.from_BMSHybrid.BMS_HYB_02.BMS_IstSpannung,from_CAN.fromHV_CAN.from_BMSHybrid.BMS_Spannung_ZwKr,from_CAN.fromHV_CAN.from_BMSHybrid.BMS_Temperatur,from_CAN.fromHV_CAN.from_BMSHybrid.BMS_Fehler_Isolation,from_CAN.fromHV_CAN.from_BMSHybrid.BMS_HYB_02.BMS_Fehler_HS_offen,from_CAN.fromHV_CAN.from_BMSHybrid.BMS_Fehler_HS_verschweisst
  Conversion  BMS_gdf : DataTypeConversion  OutDataTypeStr=boolean
  Conversion  Fehler_HS_offen : DataTypeConversion  OutDataTypeStr=boolean
  Conversion  Fehler_HS_verschweisst : DataTypeConversion  OutDataTypeStr=boolean
  Conversion  closeContactorsCmd : DataTypeConversion  OutDataTypeStr=boolean
  Conversion  contactorsClsd : DataTypeConversion  OutDataTypeStr=boolean
  Conversion  essTemp_K : DataTypeConversion  OutDataTypeStr=double
  Conversion  hvBattVolt_V : DataTypeConversion  OutDataTypeStr=double
  Conversion  hvBusVolt_V : DataTypeConversion  OutDataTypeStr=double
  Conversion  rollingAliveCnt : DataTypeConversion  OutDataTypeStr=int8
  Conversion essCur_A : DataTypeConversion  OutDataTypeStr=double
  Conversion essSOC_0_1 : DataTypeConversion  OutDataTypeStr=double
  K to C : Bias  Bias=-273.15
  Override  BMS_gdf 0_1 : Subsystem
  Override  closeContactorsCmd : Subsystem
  Override  contactorsClsd : Subsystem
  Override  essCur_A : Subsystem
  Override  essSOC_0_1 : Subsystem
  Override  essTemp_C : Subsystem
  Override  hvBattVolt_V : Subsystem
  Override  hvBusVolt_V : Subsystem
  Override  rollingAliveCnt [1_3] : Subsystem
  Override Fehler_HS_offen : Subsystem
  Override Fehler_HS_verschweisst : Subsystem
  Out1 : Outport
  wires:
  Override Fehler_HS_verschweisst/1(Out1) -> Bus Creator/11  "Fehler_HS_verschweisst"
  Conversion  Fehler_HS_verschweisst/1 -> Override Fehler_HS_verschweisst/1(In1)
  Bus Selector/10 -> Conversion  Fehler_HS_verschweisst/1  "<BMS_Fehler_HS_verschweisst>"
  Override Fehler_HS_offen/1(Out1) -> Bus Creator/10  "Fehler_HS_offen"
  Conversion  Fehler_HS_offen/1 -> Override Fehler_HS_offen/1(In1)
  Bus Selector/9 -> Conversion  Fehler_HS_offen/1  "<BMS_Fehler_HS_offen>"
  [MO_BMS_Sollmodus] -> Conversion  closeContactorsCmd/1
  Bus Selector/6 -> Conversion  hvBusVolt_V/1  "<BMS_Spannung_ZwKr>"
  Bus Selector/1 -> Conversion  rollingAliveCnt/1  "<BMS_HYB_02_BZ>"
  Bus Selector/3 -> Conversion essCur_A/1  "<BMS_IstStrom>"
  Bus Selector/4 -> Conversion essSOC_0_1/1  "<BMS_SOC>"
  Bus Selector/5 -> Conversion  hvBattVolt_V/1  "<BMS_IstSpannung>"
  Bus Selector/8 -> Conversion  BMS_gdf/1  "<BMS_Fehler_Isolation>"
  Bus Selector/7 -> Conversion  essTemp_K/1  "<BMS_Temperatur>"
  Bus Selector/2 -> Conversion  contactorsClsd/1  "<BMS_IstModus>"
  Override  BMS_gdf 0_1/1(Out1) -> Bus Creator/9  "BMS_gdf"
  Conversion  BMS_gdf/1 -> Override  BMS_gdf 0_1/1(In1)
  K to C/1 -> Override  essTemp_C/1(In1)
  Override  essTemp_C/1(Out1) -> Bus Creator/8  "essTemp_C"
  Conversion  essTemp_K/1 -> K to C/1
  Override  hvBusVolt_V/1(Out1) -> Bus Creator/7  "hvBusVolt_V"
  Override  essCur_A/1(Out1) -> Bus Creator/4  "essCur_A"
  Override  hvBattVolt_V/1(Out1) -> Bus Creator/6  "hvBattVolt_V"
  Override  essSOC_0_1/1(Out1) -> Bus Creator/5  "essSOC_0_1"
  Override  contactorsClsd/1(Out1) -> Bus Creator/3  "contactorsClsd"
  Conversion  hvBusVolt_V/1 -> Override  hvBusVolt_V/1(In1)
  Conversion  hvBattVolt_V/1 -> Override  hvBattVolt_V/1(In1)
  Conversion essSOC_0_1/1 -> Override  essSOC_0_1/1(In1)
  Conversion essCur_A/1 -> Override  essCur_A/1(In1)
  Conversion  contactorsClsd/1 -> Override  contactorsClsd/1(In1)
  Override  closeContactorsCmd/1(Out1) -> Bus Creator/2  "MO_BMS_Sollmodus [0-5]"
  Conversion  closeContactorsCmd/1 -> Override  closeContactorsCmd/1(In1)
  Bus Creator/1 -> Out1/1  "BMS_Conv"
  Override  rollingAliveCnt [1_3]/1(Out1) -> Bus Creator/1  "BMSrollingAliveCnt [123]"
  Conversion  rollingAliveCnt/1 -> Override  rollingAliveCnt [1_3]/1(In1)
  In1/1 -> Bus Selector/1

== system Hybrid_P2_Parallel/Controller/HSC/Camaro Fault Detection/Input Conversions/DriverInput_Conversions ==
  note: Driver Controls: Conversions and Override Switches
  note: SysPwrMd (EC3)
      | 0 - Off
      | 1 -  Accessory
      | 2 - Run
      | 3 - Crank Request
  In1 : Inport
  Bus Creator : BusCreator  Inputs=7
  Bus Selector : BusSelector  OutputSignals=from_Analog.Driver_APP1,from_Analog.Driver_APP2,from_CAN.fromVEH_CAN.from_BCM.BrkPdlPos,from_CAN.fromVEH_CAN.from_BCM.SysPwrMd,from_CAN.fromVEH_CAN.from_TCM.TrnsShftLvrPos,from_CAN.fromEBCAN.from_ECM.VehSpdAvgDrvn,from_Digital.SW_Regen_Disable
  Conversion  APP1 (%) : DataTypeConversion  OutDataTypeStr=double
  Conversion  APP2 (%) : DataTypeConversion  OutDataTypeStr=double
  Conversion  BPP (%) : DataTypeConversion  OutDataTypeStr=double
  Conversion  KeyPos [0_3] : DataTypeConversion  OutDataTypeStr=int8
  Conversion  V [mph] : DataTypeConversion  OutDataTypeStr=double
  Conversion PRNDL : DataTypeConversion  OutDataTypeStr=uint8
  Conversion Regen : DataTypeConversion  OutDataTypeStr=uint8
  Override  KeyPos [0_3] : Subsystem
  Override APP (%) : Subsystem
  Override APP (%)1 : Subsystem
  Override BPP (%) : Subsystem
  Override PRNDL : Subsystem
  Override Regen : Subsystem
  Override V [mph] : Subsystem
  Out1 : Outport
  wires:
  Override Regen/1(Out1) -> Bus Creator/7  "SW_Regen"
  Conversion Regen/1 -> Override Regen/1(In1)
  Bus Selector/7 -> Conversion Regen/1  "<SW_Regen_Disable>"
  Override V [mph]/1(Out1) -> Bus Creator/6  "V [mph]"
  Conversion  V [mph]/1 -> Override V [mph]/1(In1)
  Bus Selector/6 -> Conversion  V [mph]/1  "<VehSpdAvgDrvn>"
  Conversion  APP2 (%)/1 -> Override APP (%)1/1(In1)
  Override APP (%)1/1(Out1) -> Bus Creator/2  "APP2[%]"
  Bus Selector/5 -> Conversion PRNDL/1  "<TrnsShftLvrPos>"
  Bus Selector/2 -> Conversion  APP2 (%)/1  "<Driver_APP2>"
  Override PRNDL/1(Out1) -> Bus Creator/5  "PRNDL"
  Conversion PRNDL/1 -> Override PRNDL/1(In1)
  Conversion  BPP (%)/1 -> Override BPP (%)/1(In1)
  Bus Creator/1 -> Out1/1  "DriverControls_Conv"
  Override  KeyPos [0_3]/1(Out1) -> Bus Creator/4  "keyPos [0_3]"
  Override BPP (%)/1(Out1) -> Bus Creator/3  "BPP [%]"
  Conversion  KeyPos [0_3]/1 -> Override  KeyPos [0_3]/1(In1)
  Bus Selector/4 -> Conversion  KeyPos [0_3]/1  "<SysPwrMd>"
  Bus Selector/3 -> Conversion  BPP (%)/1  "<BrkPdlPos>"
  Bus Selector/1 -> Conversion  APP1 (%)/1  "<Driver_APP1>"
  Override APP (%)/1(Out1) -> Bus Creator/1  "APP1 [%]"
  Conversion  APP1 (%)/1 -> Override APP (%)/1(In1)
  In1/1 -> Bus Selector/1

== system Hybrid_P2_Parallel/Controller/HSC/Camaro Fault Detection/Input Conversions/ECM_Conversions ==
  note: ECM: Input Conversions and Override Switches
      | (Engine and ECM)
  In1 : Inport
  Bus Creator : BusCreator  Inputs=6
  Bus Selector : BusSelector  OutputSignals=from_CAN.fromEBCAN.from_ECM.PlatEngSpdCmdStARC,from_CAN.fromEBCAN.from_ECM.EngSpd,from_CAN.fromEBCAN.from_ECM.EngCltTmp,from_CAN.fromEBCAN.from_ECM.EngRunAtv,from_CAN.fromEBCAN.from_ECM.EngActStdyStTorq
  Conversion  ECMTrqCmd_Nm : DataTypeConversion  OutDataTypeStr=double
  Conversion  EngActStdyStTorq_Nm : DataTypeConversion  OutDataTypeStr=double
  Conversion  EngRunAtv : DataTypeConversion  OutDataTypeStr=boolean
  Conversion  Engine_Speed_rpm : DataTypeConversion  OutDataTypeStr=double
  Conversion  Engine_Temp[DegC] : DataTypeConversion  OutDataTypeStr=double
  Conversion  rollingAliveCnt : DataTypeConversion  OutDataTypeStr=int8
  Memory : Memory
  Override  ECMTrqCmd_Nm : Subsystem
  Override  ECMrollingAliveCnt : Subsystem
  Override  EngActStdyStTorq_Nm : Subsystem
  Override  EngRunAtv : Subsystem
  Override  EngineSpeed_rpm : Subsystem
  Override  Engine_Temp[DegC] : Subsystem
  Out1 : Outport
  wires:
  Memory/1 -> Conversion  ECMTrqCmd_Nm/1
  [AxlEngTrqCmd] -> Memory/1
  Bus Selector/1 -> Conversion  rollingAliveCnt/1  "<PlatEngSpdCmdStARC>"
  Override  EngActStdyStTorq_Nm/1(Out1) -> Bus Creator/6  "EngActStdyStTorq_Nm"
  Override  EngRunAtv/1(Out1) -> Bus Creator/5  "EngRunAtv"
  Override  Engine_Temp[DegC]/1(Out1) -> Bus Creator/4  "Engine_Temp[DegC]"
  Conversion  EngActStdyStTorq_Nm/1 -> Override  EngActStdyStTorq_Nm/1(In1)
  Conversion  EngRunAtv/1 -> Override  EngRunAtv/1(In1)
  Conversion  Engine_Temp[DegC]/1 -> Override  Engine_Temp[DegC]/1(In1)
  Bus Selector/5 -> Conversion  EngActStdyStTorq_Nm/1  "<EngActStdyStTorq>"
  Bus Selector/4 -> Conversion  EngRunAtv/1  "<EngRunAtv>"
  Bus Selector/3 -> Conversion  Engine_Temp[DegC]/1  "<EngCltTmp>"
  Override  EngineSpeed_rpm/1(Out1) -> Bus Creator/3  "EngineSpeed_rpm"
  Conversion  Engine_Speed_rpm/1 -> Override  EngineSpeed_rpm/1(In1)
  Bus Selector/2 -> Conversion  Engine_Speed_rpm/1  "<EngSpd>"
  Conversion  ECMTrqCmd_Nm/1 -> Override  ECMTrqCmd_Nm/1(In1)
  Override  ECMTrqCmd_Nm/1(Out1) -> Bus Creator/2  "ECMTrqCmd_Nm"
  Bus Creator/1 -> Out1/1  "ECM_Conv"
  Override  ECMrollingAliveCnt/1(Out1) -> Bus Creator/1  "ECMrollingAliveCnt [123]"
  Conversion  rollingAliveCnt/1 -> Override  ECMrollingAliveCnt/1(In1)
  In1/1 -> Bus Selector/1

== system Hybrid_P2_Parallel/Controller/HSC/Camaro Fault Detection/Input Conversions/TCM_Conversions ==
  note: TCM: Input Conversions and Override Switches
      | (Transmission Control Module)
  In1 : Inport
  Bus Creator : BusCreator  Inputs=4
  Bus Selector : BusSelector  OutputSignals=from_CAN.fromVEH_CAN.from_TCM.TrnsShftLvrPos,from_CAN.fromVEH_CAN.from_TCM.TransEstGear,from_CAN.fromVEH_CAN.from_TCM.TrnsTrqCnvCltCmndMd
  Conversion  LockupCmd : DataTypeConversion  OutDataTypeStr=boolean
  Conversion  LvrPosTrnsShft : DataTypeConversion  OutDataTypeStr=int8
  Conversion  TransEstGear : DataTypeConversion  OutDataTypeStr=int8
  Conversion  rollingAliveCnt : DataTypeConversion  OutDataTypeStr=int8
  Override  LockupCmd : Subsystem
  "Override  LvrPosTrnsShft " : Subsystem
  Override  TransEstGear : Subsystem
  Override  rollingAliveCnt [123] : Subsystem
  TCM_RollinAliveCounter : Subsystem
  Out1 : Outport
  wires:
  TCM_RollinAliveCounter/1(Out1) -> Conversion  rollingAliveCnt/1
  In1/1 -> Bus Selector/1
  Conversion  rollingAliveCnt/1 -> Override  rollingAliveCnt [123]/1(In1)
  Override  rollingAliveCnt [123]/1(Out1) -> Bus Creator/1  "TCMrollingAliveCnt [123]"
  Bus Creator/1 -> Out1/1  "TCM_Conv"
  Bus Selector/1 -> Conversion  LvrPosTrnsShft/1  "<TrnsShftLvrPos>"
  "Override  LvrPosTrnsShft "/1(Out1) -> Bus Creator/2  "LvrPosTrnsShft"
  Conversion  LvrPosTrnsShft/1 -> "Override  LvrPosTrnsShft "/1(In1)
  Bus Selector/2 -> Conversion  TransEstGear/1  "<TransEstGear>"
  Conversion  TransEstGear/1 -> Override  TransEstGear/1(In1)
  Override  TransEstGear/1(Out1) -> Bus Creator/3  "TransEstGear"
  Bus Selector/3 -> Conversion  LockupCmd/1  "<TrnsTrqCnvCltCmndMd>"
  Conversion  LockupCmd/1 -> Override  LockupCmd/1(In1)
  Override  LockupCmd/1(Out1) -> Bus Creator/4  "LockupCmd_0_1"

== system Hybrid_P2_Parallel/Controller/HSC/Camaro Fault Detection/Signal Diagnostic/Driver Signal Diagnostic ==
  note: Driver Controls : Signal Diagnostic
  Sensors1 : Inport
  APP_Crosscheck : Subsystem
  AccPedalValidity : Stateflow chart  TreatAsAtomicUnit=on
  AccPedalValidity1 : Stateflow chart  TreatAsAtomicUnit=on
  BPP_faild_ovrd : Constant  Value=0  OutDataTypeStr=boolean
  BrakeFailureDetection : Subsystem
  Bus Creator : BusCreator  Inputs=7
  Bus Selector : BusSelector  OutputSignals=DriverControls_Conv.APP1 [%],DriverControls_Conv.APP2[%],DriverControls_Conv.BPP [%],DriverControls_Conv.V [mph],DriverControls_Conv.keyPos [0_3],DriverControls_Conv.PRNDL
  ClearAPP1fault : Constant  Value=0
  ClearAPP2fault : Constant  Value=0
  Constant2 : Constant  Value=0
  Constant3 : Constant  OutDataTypeStr=boolean
  Conversion  APP1 (%)1 : DataTypeConversion  OutDataTypeStr=boolean
  Conversion  APP1 (%)2 : DataTypeConversion
  Conversion  APP1 (%)3 : DataTypeConversion
  Drv_APP1_valid_ovrd : Constant  Value=0  OutDataTypeStr=boolean
  Drv_APP2_valid_ovrd : Constant  Value=0  OutDataTypeStr=boolean
  Interval Test : simulink/Logic and Bit Operations/Interval Test  IntervalClosedRight=on  uplimit=100  IntervalClosedLeft=on  lowlimit=0  OutDataTypeStr=boolean
  Interval Test1 : simulink/Logic and Bit Operations/Interval Test  IntervalClosedRight=on  uplimit=3  IntervalClosedLeft=on  lowlimit=0  OutDataTypeStr=boolean
  Interval Test2 : simulink/Logic and Bit Operations/Interval Test  IntervalClosedRight=on  uplimit=4  IntervalClosedLeft=on  lowlimit=0  OutDataTypeStr=boolean
  Latch : Subsystem
  Latch1 : Subsystem
  Logical Operator1 : Logic  AllPortsSameDT=off  OutDataTypeStr=boolean
  Logical Operator5 : Logic  Operator=OR  AllPortsSameDT=off  OutDataTypeStr=boolean
  Logical Operator6 : Logic  Operator=OR  AllPortsSameDT=off  OutDataTypeStr=boolean
  Pulse Generator : DiscretePulseGenerator  PulseType=Time based  Period=0.1  PulseWidth=10
  Scope : Scope
  Driver_SigDiag : Outport
  wires:
  Pulse Generator/1 -> Scope/1, BrakeFailureDetection/Trigger
  BPP_faild_ovrd/1 -> Logical Operator1/1
  Latch1/1(Out1) -> Logical Operator1/2  "Brake_Failed"
  Logical Operator1/1 -> Conversion  APP1 (%)2/1  "Brake_Failed"
  Latch/1(Drv_APP_Agree) -> Conversion  APP1 (%)3/1  "Drv_APP_Agree"
  Interval Test1/1 -> Bus Creator/6  "Drv_KeyPos_[0 3]_SigValid"
  Conversion  APP1 (%)2/1 -> Bus Creator/5  "Brake_Failed"
  Conversion  APP1 (%)3/1 -> Bus Creator/3  "Drv_APP_Agree"
  AccPedalValidity/1(signalValid) -> Logical Operator6/2  "Drv_APP1_[%]_SigValid"
  Drv_APP1_valid_ovrd/1 -> Logical Operator6/1
  AccPedalValidity1/1(signalValid) -> Logical Operator5/2  "Drv_APP2_[%]_SigValid"
  Drv_APP2_valid_ovrd/1 -> Logical Operator5/1
  Interval Test2/1 -> Bus Creator/7  "Drv_PRNDL_SigValid"
  BrakeFailureDetection/1(DecelFail) -> Latch1/1(In1)  "Brake_Failed"
  Conversion  APP1 (%)1/1 -> Latch1/2(In2)
  Constant2/1 -> Conversion  APP1 (%)1/1
  Bus Selector/4 -> BrakeFailureDetection/2(VehSpeed)  "<V [mph]>"
  APP_Crosscheck/1(Out1) -> Latch/1(In1)  "Drv_APP_Agree"
  Constant3/1 -> Latch/2(In2)
  Bus Selector/6 -> Interval Test2/1  "<PRNDL>"
  Bus Creator/1 -> Driver_SigDiag/1  "Driver_SignalDiag"
  Logical Operator5/1 -> Bus Creator/2  "Drv_APP2_[%]_SigValid"
  Interval Test/1 -> Bus Creator/4  "Drv_BPP_[%]_SigValid"
  Logical Operator6/1 -> Bus Creator/1  "Drv_APP1_[%]_SigValid"
  Bus Selector/5 -> Interval Test1/1  "<keyPos [0_3]>"
  Bus Selector/3 -> BrakeFailureDetection/1(BPP), Interval Test/1  "<BPP [%]>"
  ClearAPP2fault/1 -> AccPedalValidity1/1(clearFaults)
  ClearAPP1fault/1 -> AccPedalValidity/1(clearFaults)
  Bus Selector/2 -> APP_Crosscheck/2(In2), AccPedalValidity1/2(signalValue)  "<APP2[%]>"
  Bus Selector/1 -> APP_Crosscheck/1(In1), AccPedalValidity/2(signalValue)  "<APP1 [%]>"
  Sensors1/1 -> Bus Selector/1
